simulink model "Furnace"  (R2020a)
settings: Solver=ode15s  StartTime=0  StopTime=27000  FixedStep=0.1  MaxStep=20  MinStep=1e-13  RelTol=1e-08  AbsTol=1e-09
undefined symbols (not defined in the file): agnostic_lqe_params, cont_reg, disturbance_type, F_aI_pid, F_aII_pid, input_type, k, lqe_params, LQR_params, LQRAgnostic_params, MPC_type, MPCDiscrete_function_parameters, MPCDiscreteAgnostic_function_parameters, MPCDiscreteDiffIntegralAgnostic_function_parameters, original_LQR_params, output_type, reg, single_butter_ss
libraries: simulink x35, cstblocks x10, mpclib x3
(part 1 of 8)
settings Model: Creator=elisam  LastModifiedBy=jorn
settings SolverCC: MaxConsecutiveZCs=10000  ZeroCrossAlgorithm=Adaptive
settings DataIOCC: FinalStateName=ss_state_out  InitialState=ss_state  LoadInitialState=on  SaveFinalState=on  SaveOperatingPoint=on  SaveFormat=Array  SaveOutput=off  DSMLogging=off  ReturnWorkspaceOutputs=off
settings OptimizationCC: BlockReduction=off  EfficientMapNaN2IntZero=off  SimCompilerOptimization=on
settings DebuggingCC: AlgebraicLoopMsg=error  ArtificialAlgebraicLoopMsg=error  UnconnectedInputMsg=none  UnconnectedOutputMsg=none  UnconnectedLineMsg=none  PregeneratedLibrarySubsystemCodeDiagnostic=none  ArithmeticOperatorsInVariantConditions=warning
settings HardwareCC: TargetBitPerLong=64  TargetBitPerPointer=64  TargetBitPerSizeT=64  TargetBitPerPtrDiffT=64  TargetLongLongMode=on  TargetIntDivRoundTo=Zero  TargetEndianess=LittleEndian  TargetWordSize=64  TargetHWDeviceType=MATLAB Host  ProdEqTarget=off
settings SFSimCC: SimUseLocalCustomCode=off  CustomCodeUndefinedFunction=UseInterfaceOnly
settings CodeAppCC: MaxIdLength=128
settings GRTTargetCC: CombineOutputUpdateFcns=off  GRTInterface=on

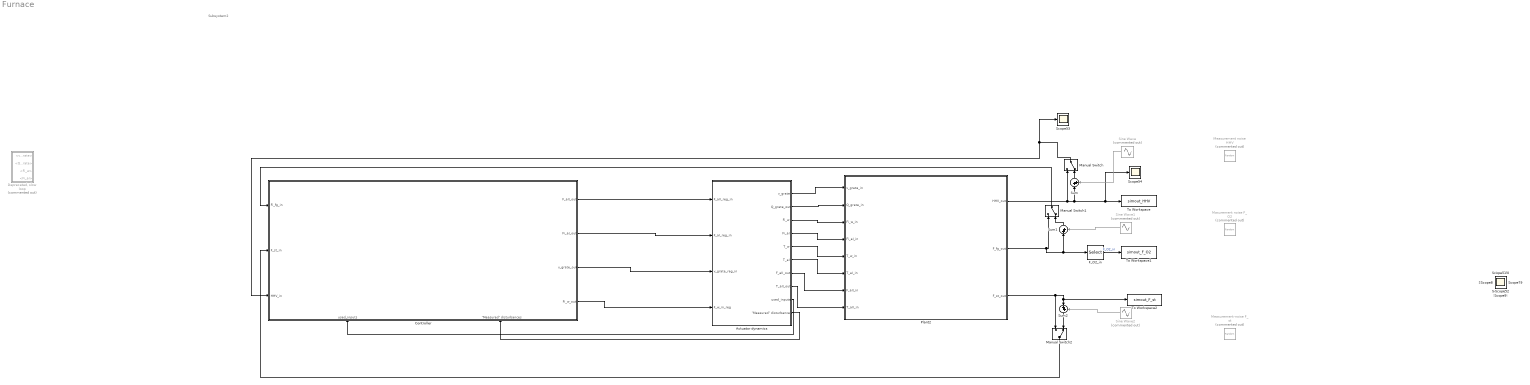
== system Furnace ==
  note: Subsystem2
  Actuator dynamics : Subsystem
  Controller : Subsystem
      settings: PortSchema="{\"entries\":[{\"content\":{\"sides\":[{\"content\":{\"connectorIds\":[\"In1\",\"In2\",\"In3\"]},\"type\":\"ConnectorPlacement.EquallySpacedRectSide\",\"uuid\":\"9212388b-0233-4c0d-abf7-b4aac7804a1a\"},{\"content\":{\"connectorIds\":[\"Out1\",\"Out2\",\"Out3\",\"Out4\"],\"side\":\"RIGHT\"},\"type\":\"ConnectorPlacement.EquallySpacedRectSide\",\"uuid\":\"ec9f57cf-6c7e-4926-bff7-17ce1d99a11a\"},{\"content\":{\"connectorIds\":[],\"side\":\"TOP\"},\"type\":\"ConnectorPlacement.EquallySpacedRectSide\",\"uuid\":\"f3c30994-927b-4377-92d1-6db743f01150\"},{\"content\":{\"connectorIds\":[\"In4\",\"In5\"],\"side\":\"BOTTOM\"},\"type\":\"ConnectorPlacement.EquallySpacedRectSide\",\"uuid\":\"c1a92049-b704-4e72-9e8e-c3f5af65781d\"}]},\"type\":\"ConnectorPlacement.EquallySpacedConnector\",\"uuid\":\"4dfd1ddf-42df-430c-9ebe-da49fca051ac\"}],\"packageUris\":[\"http://schema.mathworks.com/mf0/Connector/19700101\"],\"version\":\"1.0\"}"
  "Deprecated, slow loop" : Subsystem  Commented=on
  F_O2_in : Selector  InputPortWidth=12  IndexOptions=Index vector (dialog)  Indices=[4]  OutputSizes=1
  Manual Switch : ManualSwitch  CurrentSetting=0
  Manual Switch1 : ManualSwitch  CurrentSetting=0
  Manual Switch2 : ManualSwitch  CurrentSetting=0
  Masurement noise F_O2 : RandomNumber  Commented=on  Variance=reg.include_noise*reg.sp_F_O2*1e-3  Seed=2  SampleTime=1
  Measurement noise HHV : RandomNumber  Commented=on  Variance=reg.include_noise*reg.sp_HHV * 1e-3  Seed=1  SampleTime=1
  Measurement-noise F_st : RandomNumber  Commented=on  Variance=reg.include_noise*reg.sp_F_st* 1e-3  Seed=3  SampleTime=1
  Plant2 : Subsystem
  Scope{,1..54} (55 alike) : Scope
  Sine Wave : Sin  Commented=on  Amplitude=reg.include_noise * 1e-3  SampleTime=0
  Sine Wave1 : Sin  Commented=on  Amplitude=reg.include_noise * 1e-3  SampleTime=0
  Sine Wave2 : Sin  Commented=on  Amplitude=reg.include_noise * 1e-3  SampleTime=0
  Sum : Sum  Inputs=|++
  Sum1 : Sum  Inputs=|++
  Sum2 : Sum  Inputs=|++
  To Workspace : ToWorkspace  VariableName=simout_HHV  SaveFormat=Timeseries  SampleTime=-1
  To Workspace1 : ToWorkspace  VariableName=simout_F_O2  SaveFormat=Timeseries  SampleTime=-1
  To Workspace2 : ToWorkspace  VariableName=simout_F_st  SaveFormat=Timeseries  SampleTime=-1
  wires:
  Manual Switch2/1 -> Controller/2(F_st_in)
  Manual Switch/1 -> Scope53/1, Controller/3(HHV_in)
  Manual Switch1/1 -> Controller/1(Fi_fg_in)
  Controller/1(F_aII_out) -> Actuator dynamics/1(F_aII_reg_in)
  Controller/2(Fi_aI_out) -> Actuator dynamics/2("F_aI_reg_in ")
  Controller/3(v_grate_out) -> Actuator dynamics/3(v_grate_reg_in)
  Controller/4(Fi_w_out) -> Actuator dynamics/4(F_w_in_reg)
  Actuator dynamics/1(v_grate) -> Plant2/1(v_grate_in)
  Actuator dynamics/2(Q_grate_out) -> Plant2/2(Q_grate_in)
  Actuator dynamics/3(Fi_w) -> Plant2/3(Fi_w_in)
  Actuator dynamics/4(Fi_aI) -> Plant2/4(Fi_aI_in)
  Actuator dynamics/5(T_w) -> Plant2/5(T_w_in)
  Actuator dynamics/6(T_aI) -> Plant2/6(T_aI_in)
  Actuator dynamics/7(F_aII_out) -> Plant2/7(F_aII_in)
  Actuator dynamics/8(T_aII_out) -> Plant2/8(T_aII_in)
  F_O2_in/1 -> To Workspace1/1  "F_O2_in"
  Actuator dynamics/9(used_inputs) -> Controller/4(used_inputs)
  Sum/1 -> Manual Switch/2
  Plant2/1(HHV_out) -> Manual Switch/1, Scope54/1, To Workspace/1, Sum/1
  Plant2/2(F_fg_out) -> Manual Switch1/1, Sum1/1, F_O2_in/1
  Sum1/1 -> Manual Switch1/2
  Sum2/1 -> Manual Switch2/2
  Plant2/3(F_st_out) -> To Workspace2/1, Sum2/1, Manual Switch2/1
  Sine Wave/1 -> Sum/2
  Sine Wave1/1 -> Sum1/2
  Sine Wave2/1 -> Sum2/2
  Actuator dynamics/10("\"Measured\" disturbances") -> Controller/5("\"Measured\" disturbances")

== system Furnace/Actuator dynamics ==
  F_aII_reg_in : Inport
  "F_aI_reg_in " : Inport  Port=2
  v_grate_reg_in : Inport  Port=3
  F_w_in_reg : Inport  Port=4
  Demux : Demux  Outputs=3
  Grate speed : Subsystem
  Mux : Mux
  Mux1 : Mux  Inputs=5
  Scope : Scope
  Scope1 : Scope
  Scope2 : Scope
  Secondary air : Subsystem
      mask Display: image('airflow.jpeg');
  Waste and Primary air : Subsystem
      mask Display: image('waste_in.jpg');
  v_grate : Outport
  Q_grate_out : Outport  Port=2
  Fi_w : Outport  Port=3
  Fi_aI : Outport  Port=4
  T_w : Outport  Port=5
  T_aI : Outport  Port=6
  F_aII_out : Outport  Port=7
  T_aII_out : Outport  Port=8
  used_inputs : Outport  Port=9
  "\"Measured\" disturbances" : Outport  Port=10
  wires:
  Grate speed/1(v_grate_out) -> v_grate/1  "v_grate"
  Grate speed/2(Q_grate_out) -> Q_grate_out/1, Demux/1
  Secondary air/2(T_aII_out) -> Mux1/2, T_aII_out/1  "T_aII"
  Waste and Primary air/2(Fi_aI_out) -> Fi_aI/1  "Fi_aI"
  Waste and Primary air/3(T_w_out) -> T_w/1  "T_w"
  Waste and Primary air/1(Fi_w_out) -> Fi_w/1  "Fi_w"
  Waste and Primary air/4(T_aI_out) -> Mux1/1, T_aI/1  "T_aI"
  F_w_in_reg/1 -> Waste and Primary air/2(F_w_in_reg)
  Secondary air/1(F_aII_out) -> F_aII_out/1  "F_aII"
  v_grate_reg_in/1 -> Grate speed/1(v_grate_reg_in)
  "F_aI_reg_in "/1 -> Waste and Primary air/1("F_aI_reg_in ")
  F_aII_reg_in/1 -> Secondary air/1(F_aII_reg_in)
  Waste and Primary air/6(u_F_w) -> Mux/4, Scope/1  "u_F_w"
  Waste and Primary air/5(u_Fi_aI) -> Mux/2, Scope1/1  "u_F_aI"
  Secondary air/3(u_F_aII) -> Mux/1, Scope2/1  "u_F_aII"
  Grate speed/3(u_v_grate) -> Mux/3
  Mux/1 -> used_inputs/1
  Mux1/1 -> "\"Measured\" disturbances"/1
  Demux/3 -> Mux1/5
  Demux/2 -> Mux1/4
  Demux/1 -> Mux1/3

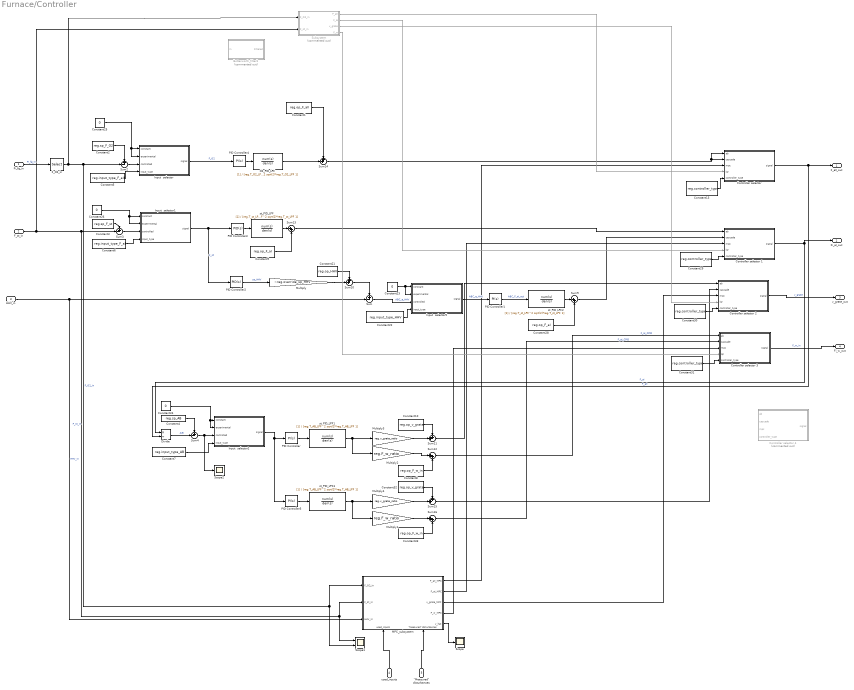
== system Furnace/Controller ==
  Fi_fg_in : Inport
  F_st_in : Inport  Port=2
  HHV_in : Inport  Port=3
  used_inputs : Inport  Port=4
  "\"Measured\" disturbances" : Inport  Port=5
  Butterworth_filter3 : Subsystem  Commented=on
  Constant1 : Constant  Value=reg.op_F_aII
  Constant10 : Constant  Value=reg.op_v_grate
  Constant{13,29..31} (4 alike) : Constant  Value=reg.controller_type
  Constant2 : Constant  Value=reg.sp_F_O2
  Constant21 : Constant  Value=reg.op_HHV
  Constant22 : Constant  Value=reg.input_type_HHV
  Constant{23..26} (4 alike) : Constant  Value=0
  Constant28 : Constant  Value=reg.op_F_aI
  Constant3 : Constant  Value=reg.sp_F_st
  Constant32 : Constant  Value=reg.op_v_grate
  Constant33 : Constant  Value=reg.op_F_w_in
  Constant4 : Constant  Value=reg.sp_AB
  Constant5 : Constant  Value=reg.input_type_F_aII
  Constant6 : Constant  Value=reg.input_type_F_aI
  Constant7 : Constant  Value=reg.input_type_AB
  Constant8 : Constant  Value=reg.op_F_w_in
  Constant9 : Constant  Value=reg.op_F_aI
  "Controller selector " : MATLAB Function  TreatAsAtomicUnit=on
  Controller selector 1 : MATLAB Function  TreatAsAtomicUnit=on
  Controller selector 2 : MATLAB Function  TreatAsAtomicUnit=on
  Controller selector 3 : MATLAB Function  TreatAsAtomicUnit=on
  Controller selector 4 : MATLAB Function  Commented=on  TreatAsAtomicUnit=on
  Divide : Product  Inputs=*/  OutMin=[-100]  OutMax=[100]
  F_O2_in : Selector  InputPortWidth=12  IndexOptions=Index vector (dialog)  Indices=[4]  OutputSizes=1
  Input  selector : MATLAB Function  TreatAsAtomicUnit=on
  Input  selector1 : MATLAB Function  TreatAsAtomicUnit=on
  Input  selector2 : MATLAB Function  TreatAsAtomicUnit=on
  Input  selector5 : MATLAB Function  TreatAsAtomicUnit=on
  MPC_subsystem : Subsystem
      settings: PortSchema="{\"entries\":[{\"content\":{\"sides\":[{\"content\":{\"connectorIds\":[\"In1\",\"In2\",\"In3\"]},\"type\":\"ConnectorPlacement.EquallySpacedRectSide\",\"uuid\":\"7a72dc7f-38c0-42c0-80ed-1e6801fa5538\"},{\"content\":{\"connectorIds\":[\"Out1\",\"Out2\",\"Out3\",\"Out4\",\"Out5\"],\"side\":\"RIGHT\"},\"type\":\"ConnectorPlacement.EquallySpacedRectSide\",\"uuid\":\"3b96338e-56f2-4c6d-b025-d8deebb787e0\"},{\"content\":{\"connectorIds\":[],\"side\":\"TOP\"},\"type\":\"ConnectorPlacement.EquallySpacedRectSide\",\"uuid\":\"204ca672-7e69-45d1-bd78-35e421377db1\"},{\"content\":{\"connectorIds\":[\"In4\",\"In5\"],\"side\":\"BOTTOM\"},\"type\":\"ConnectorPlacement.EquallySpacedRectSide\",\"uuid\":\"d178d855-840b-4794-a5e2-c07226929ecd\"}]},\"type\":\"ConnectorPlacement.EquallySpacedConnector\",\"uuid\":\"1be467ef-13fc-4acb-88f5-eb362f838469\"}],\"packageUris\":[\"http://schema.mathworks.com/mf0/Connector/19700101\"],\"version\":\"1.0\"}"
  Multiply : Gain  Gain=~reg.override_sp_HHV
  Multiply1 : Gain  Gain=reg.F_w_ratio
  Multiply2 : Gain  Gain=reg.F_w_ratio
  Multiply3 : Gain  Gain=reg.v_grate_ratio
  Multiply4 : Gain  Gain=reg.v_grate_ratio
  O2_PID_LPF : TransferFcn  Denominator=[reg.T_O2_LPF^2 sqrt(2)*reg.T_O2_LPF 1]
  PID Controller : simulink/Continuous/PID Controller  Controller=PI  Form=Parallel  TimeDomain=Continuous-time  UseExternalTs=off  SampleTime=1  IntegratorMethod=Forward Euler  FilterMethod=Forward Euler  ControllerParametersSource=internal  P=reg.Kp_AB  I=reg.Ki_AB  D=0  UseFilter=on  N=100  TunerSelectOption=Transfer Function Based (PID Tuner App)  InitialConditionSource=internal  InitialConditionForIntegrator=0  InitialConditionForFilter=0  DifferentiatorICPrevScaledInput=0  ExternalReset=none  TrackingMode=off  Kt=1  LimitOutput=off  UpperSaturationLimit=inf  LowerSaturationLimit=-inf  LinearizeAsGain=on  AntiWindupMode=none  Kb=1  POutMin=[]  POutMax=[]  IOutMin=[]  IOutMax=[]  DOutMin=[]  DOutMax=[]  NOutMin=[]  NOutMax=[]  SumOutMin=[]  SumOutMax=[]  SaturationOutMin=[]  SaturationOutMax=[]  PParamMin=[]  PParamMax=[]  IParamMin=[]  IParamMax=[]  DParamMin=[]  DParamMax=[]  NParamMin=[]  NParamMax=[]  KbParamMin=[]  KbParamMax=[]  KtParamMin=[]  KtParamMax=[]  KbOutMin=[]  KbOutMax=[]  KtOutMin=[]  KtOutMax=[]  IntegratorOutMin=[]  IntegratorOutMax=[]  FilterOutMin=[]  FilterOutMax=[]  SumI1OutMin=[]  SumI1OutMax=[]  SumI2OutMin=[]  SumI2OutMax=[]  SumI3OutMin=[]  SumI3OutMax=[]  SumI4OutMin=[]  SumI4OutMax=[]  SumDOutMin=[]  SumDOutMax=[]  DifferentiatorOutMin=[]  DifferentiatorOutMax=[]  FilterDiffOutCoefMin=[]  FilterDiffOutCoefMax=[]  ReciprocalOutMin=[]  ReciprocalOutMax=[]  SumDenOutMin=[]  SumDenOutMax=[]  SumNumOutMin=[]  SumNumOutMax=[]  DivideOutMin=[]  DivideOutMax=[]  UdiffTsProdOutMin=[]  UdiffTsProdOutMax=[]  NTsProdOutMin=[]  NTsProdOutMax=[]  UintegralTsProdOutMin=[]  UintegralTsProdOutMax=[]  UngainTsProdOutMin=[]  UngainTsProdOutMax=[]  IntegratorContinuousStateAttributes=''  IntegratorStateMustResolveToSignalObject=off  IntegratorRTWStateStorageClass=Auto  FilterContinuousStateAttributes=''  FilterStateMustResolveToSignalObject=off  FilterRTWStateStorageClass=Auto  ParallelPVariant=InternalParameters  IdealPVariant=Disabled  IVariant=InternalParameters  DVariant=Disabled  IntegratorVariant=Continuous  SatVariant=Disabled  AWVariant=Passthrough  PCopyVariant=Disabled  TRVariant=Disabled  FdbkBlocksVariant=Forward  IdealPFdbkVariant=Disabled  SatFdbkVariant=Disabled  DerivativeFilterVariant=Disabled  NVariant=Disabled  NCopyVariant=Disabled_SignalSpec  FilterICVariant=Disabled  IntegratorICVariant=InternalICs  ExternalResetVariant=Disabled  TRSumVariant=Passthrough  SumFdbkVariant=Disabled  SumVariant=Sum_PI  TsampFilterVariant=InternalTs  TsampNgainVariant=Passthrough  TsampIntegralVariant=Passthrough
  PID Controller1 : simulink/Continuous/PID Controller  Controller=PI  Form=Parallel  TimeDomain=Continuous-time  UseExternalTs=off  SampleTime=1  IntegratorMethod=Forward Euler  FilterMethod=Forward Euler  ControllerParametersSource=internal  P=reg.Kp_HHV  I=reg.Ki_HHV  D=0  UseFilter=on  N=100  TunerSelectOption=Transfer Function Based (PID Tuner App)  InitialConditionSource=internal  InitialConditionForIntegrator=0  InitialConditionForFilter=0  DifferentiatorICPrevScaledInput=0  ExternalReset=none  TrackingMode=off  Kt=1  LimitOutput=off  UpperSaturationLimit=inf  LowerSaturationLimit=-inf  LinearizeAsGain=on  AntiWindupMode=none  Kb=1  POutMin=[]  POutMax=[]  IOutMin=[]  IOutMax=[]  DOutMin=[]  DOutMax=[]  NOutMin=[]  NOutMax=[]  SumOutMin=[]  SumOutMax=[]  SaturationOutMin=[]  SaturationOutMax=[]  PParamMin=[]  PParamMax=[]  IParamMin=[]  IParamMax=[]  DParamMin=[]  DParamMax=[]  NParamMin=[]  NParamMax=[]  KbParamMin=[]  KbParamMax=[]  KtParamMin=[]  KtParamMax=[]  KbOutMin=[]  KbOutMax=[]  KtOutMin=[]  KtOutMax=[]  IntegratorOutMin=[]  IntegratorOutMax=[]  FilterOutMin=[]  FilterOutMax=[]  SumI1OutMin=[]  SumI1OutMax=[]  SumI2OutMin=[]  SumI2OutMax=[]  SumI3OutMin=[]  SumI3OutMax=[]  SumI4OutMin=[]  SumI4OutMax=[]  SumDOutMin=[]  SumDOutMax=[]  DifferentiatorOutMin=[]  DifferentiatorOutMax=[]  FilterDiffOutCoefMin=[]  FilterDiffOutCoefMax=[]  ReciprocalOutMin=[]  ReciprocalOutMax=[]  SumDenOutMin=[]  SumDenOutMax=[]  SumNumOutMin=[]  SumNumOutMax=[]  DivideOutMin=[]  DivideOutMax=[]  UdiffTsProdOutMin=[]  UdiffTsProdOutMax=[]  NTsProdOutMin=[]  NTsProdOutMax=[]  UintegralTsProdOutMin=[]  UintegralTsProdOutMax=[]  UngainTsProdOutMin=[]  UngainTsProdOutMax=[]  IntegratorContinuousStateAttributes=''  IntegratorStateMustResolveToSignalObject=off  IntegratorRTWStateStorageClass=Auto  FilterContinuousStateAttributes=''  FilterStateMustResolveToSignalObject=off  FilterRTWStateStorageClass=Auto  ParallelPVariant=InternalParameters  IdealPVariant=Disabled  IVariant=InternalParameters  DVariant=Disabled  IntegratorVariant=Continuous  SatVariant=Disabled  AWVariant=Passthrough  PCopyVariant=Disabled  TRVariant=Disabled  FdbkBlocksVariant=Forward  IdealPFdbkVariant=Disabled  SatFdbkVariant=Disabled  DerivativeFilterVariant=Disabled  NVariant=Disabled  NCopyVariant=Disabled_SignalSpec  FilterICVariant=Disabled  IntegratorICVariant=InternalICs  ExternalResetVariant=Disabled  TRSumVariant=Passthrough  SumFdbkVariant=Disabled  SumVariant=Sum_PI  TsampFilterVariant=InternalTs  TsampNgainVariant=Passthrough  TsampIntegralVariant=Passthrough
  PID Controller2 : simulink/Continuous/PID Controller  Controller=PID  Form=Parallel  TimeDomain=Continuous-time  UseExternalTs=off  SampleTime=1  IntegratorMethod=Forward Euler  FilterMethod=Forward Euler  ControllerParametersSource=internal  P=reg.Kp_st_HHV  I=reg.Ki_st_HHV  D=reg.Kd_st_HHV  UseFilter=on  N=100  TunerSelectOption=Transfer Function Based (PID Tuner App)  InitialConditionSource=internal  InitialConditionForIntegrator=0.001  InitialConditionForFilter=0  DifferentiatorICPrevScaledInput=0  ExternalReset=none  TrackingMode=off  Kt=1  LimitOutput=off  UpperSaturationLimit=inf  LowerSaturationLimit=1  LinearizeAsGain=on  AntiWindupMode=none  Kb=1  POutMin=[]  POutMax=[]  IOutMin=[]  IOutMax=[]  DOutMin=[]  DOutMax=[]  NOutMin=[]  NOutMax=[]  SumOutMin=[]  SumOutMax=[]  SaturationOutMin=[]  SaturationOutMax=[]  PParamMin=[]  PParamMax=[]  IParamMin=[]  IParamMax=[]  DParamMin=[]  DParamMax=[]  NParamMin=[]  NParamMax=[]  KbParamMin=[]  KbParamMax=[]  KtParamMin=[]  KtParamMax=[]  KbOutMin=[]  KbOutMax=[]  KtOutMin=[]  KtOutMax=[]  IntegratorOutMin=[]  IntegratorOutMax=[]  FilterOutMin=[]  FilterOutMax=[]  SumI1OutMin=[]  SumI1OutMax=[]  SumI2OutMin=[]  SumI2OutMax=[]  SumI3OutMin=[]  SumI3OutMax=[]  SumI4OutMin=[]  SumI4OutMax=[]  SumDOutMin=[]  SumDOutMax=[]  DifferentiatorOutMin=[]  DifferentiatorOutMax=[]  FilterDiffOutCoefMin=[]  FilterDiffOutCoefMax=[]  ReciprocalOutMin=[]  ReciprocalOutMax=[]  SumDenOutMin=[]  SumDenOutMax=[]  SumNumOutMin=[]  SumNumOutMax=[]  DivideOutMin=[]  DivideOutMax=[]  UdiffTsProdOutMin=[]  UdiffTsProdOutMax=[]  NTsProdOutMin=[]  NTsProdOutMax=[]  UintegralTsProdOutMin=[]  UintegralTsProdOutMax=[]  UngainTsProdOutMin=[]  UngainTsProdOutMax=[]  IntegratorContinuousStateAttributes='F_st'  IntegratorStateMustResolveToSignalObject=off  IntegratorRTWStateStorageClass=Auto  FilterContinuousStateAttributes=''  FilterStateMustResolveToSignalObject=off  FilterRTWStateStorageClass=Auto  ParallelPVariant=InternalParameters  IdealPVariant=Disabled  IVariant=InternalParameters  DVariant=InternalParameters  IntegratorVariant=Continuous  SatVariant=Disabled  AWVariant=Passthrough  PCopyVariant=Disabled  TRVariant=Disabled  FdbkBlocksVariant=Forward  IdealPFdbkVariant=Disabled  SatFdbkVariant=Disabled  DerivativeFilterVariant=ContFilter  NVariant=InternalParameters  NCopyVariant=Disabled  FilterICVariant=InternalICsFilter  IntegratorICVariant=InternalICs  ExternalResetVariant=Disabled  TRSumVariant=Passthrough  SumFdbkVariant=Disabled  SumVariant=Sum_PID  TsampFilterVariant=InternalTs  TsampNgainVariant=Passthrough  TsampIntegralVariant=Passthrough
  PID Controller3 : simulink/Continuous/PID Controller  Controller=PID  Form=Parallel  TimeDomain=Continuous-time  UseExternalTs=off  SampleTime=1  IntegratorMethod=Forward Euler  FilterMethod=Forward Euler  ControllerParametersSource=internal  P=reg.Kp_st  I=reg.Ki_st  D=reg.Kd_st  UseFilter=on  N=100  TunerSelectOption=Transfer Function Based (PID Tuner App)  InitialConditionSource=internal  InitialConditionForIntegrator=0  InitialConditionForFilter=0  DifferentiatorICPrevScaledInput=0  ExternalReset=none  TrackingMode=off  Kt=1  LimitOutput=off  UpperSaturationLimit=inf  LowerSaturationLimit=1  LinearizeAsGain=on  AntiWindupMode=none  Kb=1  POutMin=[]  POutMax=[]  IOutMin=[]  IOutMax=[]  DOutMin=[]  DOutMax=[]  NOutMin=[]  NOutMax=[]  SumOutMin=[]  SumOutMax=[]  SaturationOutMin=[]  SaturationOutMax=[]  PParamMin=[]  PParamMax=[]  IParamMin=[]  IParamMax=[]  DParamMin=[]  DParamMax=[]  NParamMin=[]  NParamMax=[]  KbParamMin=[]  KbParamMax=[]  KtParamMin=[]  KtParamMax=[]  KbOutMin=[]  KbOutMax=[]  KtOutMin=[]  KtOutMax=[]  IntegratorOutMin=[]  IntegratorOutMax=[]  FilterOutMin=[]  FilterOutMax=[]  SumI1OutMin=[]  SumI1OutMax=[]  SumI2OutMin=[]  SumI2OutMax=[]  SumI3OutMin=[]  SumI3OutMax=[]  SumI4OutMin=[]  SumI4OutMax=[]  SumDOutMin=[]  SumDOutMax=[]  DifferentiatorOutMin=[]  DifferentiatorOutMax=[]  FilterDiffOutCoefMin=[]  FilterDiffOutCoefMax=[]  ReciprocalOutMin=[]  ReciprocalOutMax=[]  SumDenOutMin=[]  SumDenOutMax=[]  SumNumOutMin=[]  SumNumOutMax=[]  DivideOutMin=[]  DivideOutMax=[]  UdiffTsProdOutMin=[]  UdiffTsProdOutMax=[]  NTsProdOutMin=[]  NTsProdOutMax=[]  UintegralTsProdOutMin=[]  UintegralTsProdOutMax=[]  UngainTsProdOutMin=[]  UngainTsProdOutMax=[]  IntegratorContinuousStateAttributes='F_st'  IntegratorStateMustResolveToSignalObject=off  IntegratorRTWStateStorageClass=Auto  FilterContinuousStateAttributes=''  FilterStateMustResolveToSignalObject=off  FilterRTWStateStorageClass=Auto  ParallelPVariant=InternalParameters  IdealPVariant=Disabled  IVariant=InternalParameters  DVariant=InternalParameters  IntegratorVariant=Continuous  SatVariant=Disabled  AWVariant=Passthrough  PCopyVariant=Disabled  TRVariant=Disabled  FdbkBlocksVariant=Forward  IdealPFdbkVariant=Disabled  SatFdbkVariant=Disabled  DerivativeFilterVariant=ContFilter  NVariant=InternalParameters  NCopyVariant=Disabled  FilterICVariant=InternalICsFilter  IntegratorICVariant=InternalICs  ExternalResetVariant=Disabled  TRSumVariant=Passthrough  SumFdbkVariant=Disabled  SumVariant=Sum_PID  TsampFilterVariant=InternalTs  TsampNgainVariant=Passthrough  TsampIntegralVariant=Passthrough
  PID Controller4 : simulink/Continuous/PID Controller  Controller=PI  Form=Parallel  TimeDomain=Continuous-time  UseExternalTs=off  SampleTime=1  IntegratorMethod=Forward Euler  FilterMethod=Forward Euler  ControllerParametersSource=internal  P=reg.Kp_O2  I=reg.Ki_O2  D=0  UseFilter=on  N=100  TunerSelectOption=Transfer Function Based (PID Tuner App)  InitialConditionSource=internal  InitialConditionForIntegrator=0.001  InitialConditionForFilter=0  DifferentiatorICPrevScaledInput=0  ExternalReset=none  TrackingMode=off  Kt=1  LimitOutput=off  UpperSaturationLimit=inf  LowerSaturationLimit=1  LinearizeAsGain=on  AntiWindupMode=none  Kb=1  POutMin=[]  POutMax=[]  IOutMin=[]  IOutMax=[]  DOutMin=[]  DOutMax=[]  NOutMin=[]  NOutMax=[]  SumOutMin=[]  SumOutMax=[]  SaturationOutMin=[]  SaturationOutMax=[]  PParamMin=[]  PParamMax=[]  IParamMin=[]  IParamMax=[]  DParamMin=[]  DParamMax=[]  NParamMin=[]  NParamMax=[]  KbParamMin=[]  KbParamMax=[]  KtParamMin=[]  KtParamMax=[]  KbOutMin=[]  KbOutMax=[]  KtOutMin=[]  KtOutMax=[]  IntegratorOutMin=[]  IntegratorOutMax=[]  FilterOutMin=[]  FilterOutMax=[]  SumI1OutMin=[]  SumI1OutMax=[]  SumI2OutMin=[]  SumI2OutMax=[]  SumI3OutMin=[]  SumI3OutMax=[]  SumI4OutMin=[]  SumI4OutMax=[]  SumDOutMin=[]  SumDOutMax=[]  DifferentiatorOutMin=[]  DifferentiatorOutMax=[]  FilterDiffOutCoefMin=[]  FilterDiffOutCoefMax=[]  ReciprocalOutMin=[]  ReciprocalOutMax=[]  SumDenOutMin=[]  SumDenOutMax=[]  SumNumOutMin=[]  SumNumOutMax=[]  DivideOutMin=[]  DivideOutMax=[]  UdiffTsProdOutMin=[]  UdiffTsProdOutMax=[]  NTsProdOutMin=[]  NTsProdOutMax=[]  UintegralTsProdOutMin=[]  UintegralTsProdOutMax=[]  UngainTsProdOutMin=[]  UngainTsProdOutMax=[]  IntegratorContinuousStateAttributes='F_st'  IntegratorStateMustResolveToSignalObject=off  IntegratorRTWStateStorageClass=Auto  FilterContinuousStateAttributes=''  FilterStateMustResolveToSignalObject=off  FilterRTWStateStorageClass=Auto  ParallelPVariant=InternalParameters  IdealPVariant=Disabled  IVariant=InternalParameters  DVariant=Disabled  IntegratorVariant=Continuous  SatVariant=Disabled  AWVariant=Passthrough  PCopyVariant=Disabled  TRVariant=Disabled  FdbkBlocksVariant=Forward  IdealPFdbkVariant=Disabled  SatFdbkVariant=Disabled  DerivativeFilterVariant=Disabled  NVariant=Disabled  NCopyVariant=Disabled_SignalSpec  FilterICVariant=Disabled  IntegratorICVariant=InternalICs  ExternalResetVariant=Disabled  TRSumVariant=Passthrough  SumFdbkVariant=Disabled  SumVariant=Sum_PI  TsampFilterVariant=InternalTs  TsampNgainVariant=Passthrough  TsampIntegralVariant=Passthrough
  PID Controller5 : simulink/Continuous/PID Controller  Controller=PI  Form=Parallel  TimeDomain=Continuous-time  UseExternalTs=off  SampleTime=1  IntegratorMethod=Forward Euler  FilterMethod=Forward Euler  ControllerParametersSource=internal  P=reg.Kp_AB_HHV  I=reg.Ki_AB_HHV  D=0  UseFilter=on  N=100  TunerSelectOption=Transfer Function Based (PID Tuner App)  InitialConditionSource=internal  InitialConditionForIntegrator=0  InitialConditionForFilter=0  DifferentiatorICPrevScaledInput=0  ExternalReset=none  TrackingMode=off  Kt=1  LimitOutput=off  UpperSaturationLimit=inf  LowerSaturationLimit=-inf  LinearizeAsGain=on  AntiWindupMode=none  Kb=1  POutMin=[]  POutMax=[]  IOutMin=[]  IOutMax=[]  DOutMin=[]  DOutMax=[]  NOutMin=[]  NOutMax=[]  SumOutMin=[]  SumOutMax=[]  SaturationOutMin=[]  SaturationOutMax=[]  PParamMin=[]  PParamMax=[]  IParamMin=[]  IParamMax=[]  DParamMin=[]  DParamMax=[]  NParamMin=[]  NParamMax=[]  KbParamMin=[]  KbParamMax=[]  KtParamMin=[]  KtParamMax=[]  KbOutMin=[]  KbOutMax=[]  KtOutMin=[]  KtOutMax=[]  IntegratorOutMin=[]  IntegratorOutMax=[]  FilterOutMin=[]  FilterOutMax=[]  SumI1OutMin=[]  SumI1OutMax=[]  SumI2OutMin=[]  SumI2OutMax=[]  SumI3OutMin=[]  SumI3OutMax=[]  SumI4OutMin=[]  SumI4OutMax=[]  SumDOutMin=[]  SumDOutMax=[]  DifferentiatorOutMin=[]  DifferentiatorOutMax=[]  FilterDiffOutCoefMin=[]  FilterDiffOutCoefMax=[]  ReciprocalOutMin=[]  ReciprocalOutMax=[]  SumDenOutMin=[]  SumDenOutMax=[]  SumNumOutMin=[]  SumNumOutMax=[]  DivideOutMin=[]  DivideOutMax=[]  UdiffTsProdOutMin=[]  UdiffTsProdOutMax=[]  NTsProdOutMin=[]  NTsProdOutMax=[]  UintegralTsProdOutMin=[]  UintegralTsProdOutMax=[]  UngainTsProdOutMin=[]  UngainTsProdOutMax=[]  IntegratorContinuousStateAttributes=''  IntegratorStateMustResolveToSignalObject=off  IntegratorRTWStateStorageClass=Auto  FilterContinuousStateAttributes=''  FilterStateMustResolveToSignalObject=off  FilterRTWStateStorageClass=Auto  ParallelPVariant=InternalParameters  IdealPVariant=Disabled  IVariant=InternalParameters  DVariant=Disabled  IntegratorVariant=Continuous  SatVariant=Disabled  AWVariant=Passthrough  PCopyVariant=Disabled  TRVariant=Disabled  FdbkBlocksVariant=Forward  IdealPFdbkVariant=Disabled  SatFdbkVariant=Disabled  DerivativeFilterVariant=Disabled  NVariant=Disabled  NCopyVariant=Disabled_SignalSpec  FilterICVariant=Disabled  IntegratorICVariant=InternalICs  ExternalResetVariant=Disabled  TRSumVariant=Passthrough  SumFdbkVariant=Disabled  SumVariant=Sum_PI  TsampFilterVariant=InternalTs  TsampNgainVariant=Passthrough  TsampIntegralVariant=Passthrough
  Scope : Scope
  Scope1 : Scope  NumInputPorts=2
  Scope2 : Scope
  Subsystem : Subsystem  Commented=on
  Sum{,2..4} (4 alike) : Sum  Inputs=+-|
  Sum{10..11,14..15} (4 alike) : Sum  Inputs=++|
  Sum{9,12..13,16} (4 alike) : Sum  Inputs=|++
  st_PID_LPF : TransferFcn  Denominator=[reg.T_st_LPF^2 sqrt(2)*reg.T_st_LPF 1]
  st_PID_LPF1 : TransferFcn  Denominator=[reg.T_AB_LPF^2 sqrt(2)*reg.T_AB_LPF 1]
  st_PID_LPF2 : TransferFcn  Denominator=[reg.T_st_LPF^2 sqrt(2)*reg.T_st_LPF 1]
  st_PID_LPF3 : TransferFcn  Denominator=[reg.T_AB_LPF^2 sqrt(2)*reg.T_AB_LPF 1]
  F_aII_out : Outport  VectorParamsAs1DForOutWhenUnconnected=off
  Fi_aI_out : Outport  Port=2  VectorParamsAs1DForOutWhenUnconnected=off
  v_grate_out : Outport  Port=3  VectorParamsAs1DForOutWhenUnconnected=off
  Fi_w_out : Outport  Port=4  VectorParamsAs1DForOutWhenUnconnected=off
  wires:
  Input  selector/1(signal) -> PID Controller4/1  "F_O2"
  Constant7/1 -> Input  selector2/4(input_type)
  Constant5/1 -> Input  selector/4(input_type)
  Constant4/1 -> Sum4/1
  Fi_fg_in/1 -> F_O2_in/1  "Fi_fg_in"
  Constant2/1 -> Sum2/1
  F_st_in/1 -> Subsystem/2(F_st_in), Scope1/1, MPC_subsystem/2(F_st_in), Sum3/2  "F_st_in"
  Constant3/1 -> Sum3/1
  F_O2_in/1 -> Subsystem/1(F_O2_in), Scope1/2, MPC_subsystem/1(F_O2_in), Sum2/2  "F_O2_in"
  PID Controller4/1 -> O2_PID_LPF/1
  Sum14/1 -> "Controller selector "/1(ab), "Controller selector "/2(cascade)
  PID Controller3/1 -> st_PID_LPF/1
  Sum13/1 -> Controller selector 1/1(ab)
  Constant8/1 -> Sum12/2
  PID Controller/1 -> st_PID_LPF1/1
  Sum11/1 -> Controller selector 2/1(ab)
  Multiply2/1 -> Sum12/1
  Constant10/1 -> Sum11/1
  st_PID_LPF/1 -> Sum13/1
  st_PID_LPF1/1 -> Multiply2/1, Multiply3/1
  "Controller selector "/1(signal) -> Divide/2, F_aII_out/1  "F_aII"
  Controller selector 1/1(signal) -> Fi_aI_out/1, Divide/1  "F_aI"
  Controller selector 2/1(signal) -> v_grate_out/1  "v_grate"
  Controller selector 3/1(signal) -> Fi_w_out/1  "F_w_in"
  HHV_in/1 -> MPC_subsystem/3(HHV_in), Sum/2  "HHV_in"
  Input  selector5/1(signal) -> PID Controller1/1  "ABC_e_HHV"
  Constant22/1 -> Input  selector5/4(input_type)
  Sum/1 -> Input  selector5/3(controlled)  "ABC_e_HHV"
  Constant23/1 -> Input  selector5/2(experimental), Input  selector5/1(constant)
  Divide/1 -> Sum4/2  "A/B"
  Sum4/1 -> Scope2/1, Input  selector2/3(controlled)
  Input  selector2/1(signal) -> PID Controller5/1, PID Controller/1
  Constant24/1 -> Input  selector2/2(experimental), Input  selector2/1(constant)
  Sum2/1 -> Input  selector/3(controlled)
  Constant25/1 -> Input  selector/2(experimental), Input  selector/1(constant)
  Sum3/1 -> Input  selector1/3(controlled)
  Constant6/1 -> Input  selector1/4(input_type)
  Constant26/1 -> Input  selector1/2(experimental), Input  selector1/1(constant)
  Input  selector1/1(signal) -> PID Controller3/1, PID Controller2/1  "F_st"
  Sum12/1 -> Controller selector 3/1(ab)  "F_aI_CPID"
  PID Controller1/1 -> st_PID_LPF2/1  "ABC_F_aI_out"
  Sum9/1 -> Controller selector 1/2(cascade)
  PID Controller2/1 -> Multiply/1  "sp_HHV"
  Multiply/1 -> Sum10/2
  Constant21/1 -> Sum10/1
  Sum10/1 -> Sum/1
  st_PID_LPF2/1 -> Sum9/1
  Constant28/1 -> Sum9/2
  Constant9/1 -> Sum13/2
  O2_PID_LPF/1 -> Sum14/2
  Constant1/1 -> Sum14/1
  Constant13/1 -> "Controller selector "/5(controller_type)
  Constant29/1 -> Controller selector 1/5(controller_type)
  Constant30/1 -> Controller selector 2/5(controller_type)
  Constant31/1 -> Controller selector 3/5(controller_type)
  st_PID_LPF3/1 -> Multiply1/1, Multiply4/1
  PID Controller5/1 -> st_PID_LPF3/1
  Constant33/1 -> Sum16/2
  Constant32/1 -> Sum15/1
  Multiply1/1 -> Sum16/1
  Sum15/1 -> Controller selector 2/2(cascade)
  Sum16/1 -> Controller selector 3/2(cascade)  "F_aI_CPID"
  Multiply3/1 -> Sum11/2
  Multiply4/1 -> Sum15/2
  MPC_subsystem/1(F_aII_MPC) -> "Controller selector "/3(mpc)
  MPC_subsystem/2(F_aI_MPC) -> Controller selector 1/3(mpc)
  MPC_subsystem/3(v_grate_MPC) -> Controller selector 2/3(mpc)
  MPC_subsystem/4(F_w_MPC) -> Controller selector 3/3(mpc)
  MPC_subsystem/5(y_hat) -> Scope/1
  used_inputs/1 -> MPC_subsystem/4(used_inputs)
  "\"Measured\" disturbances"/1 -> MPC_subsystem/5("\"Measured\" disturbances")
  Subsystem/1(F_aII) -> "Controller selector "/4(lqr)
  Subsystem/2(F_aI) -> Controller selector 1/4(lqr)
  Subsystem/3(v_grate) -> Controller selector 2/4(lqr)
  Subsystem/4(F_w) -> Controller selector 3/4(lqr)

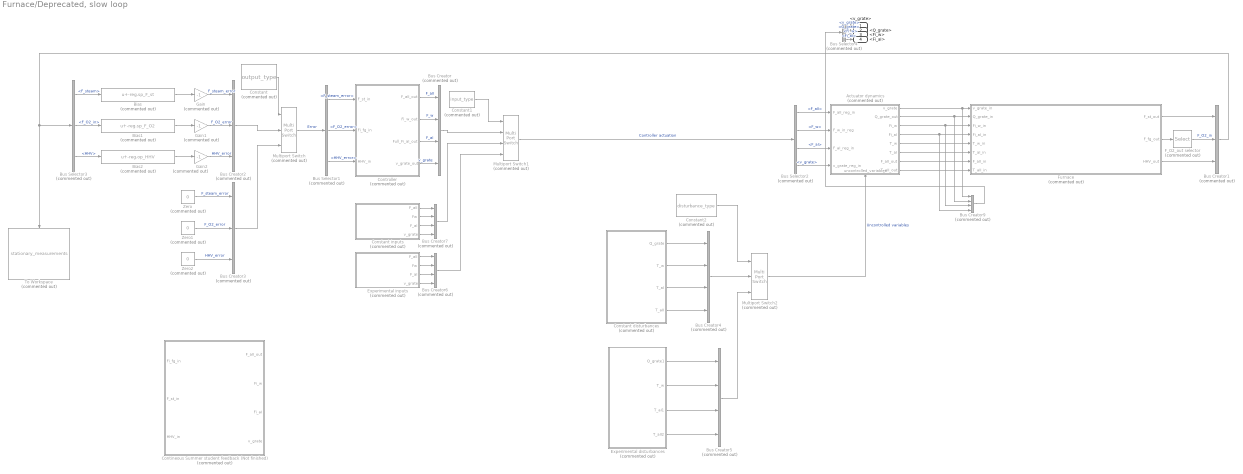
== system Furnace/Deprecated, slow loop ==
  Actuator dynamics : Subsystem  Commented=on
      settings: PortSchema="{\"entries\":[{\"content\":{\"sides\":[{\"content\":{\"connectorIds\":[\"In1\",\"In2\",\"In3\",\"In4\"]},\"type\":\"ConnectorPlacement.EquallySpacedRectSide\",\"uuid\":\"9c70279c-77f9-448c-8401-2f06341e8012\"},{\"content\":{\"connectorIds\":[\"Out1\",\"Out2\",\"Out3\",\"Out4\",\"Out5\",\"Out6\",\"Out7\",\"Out8\"],\"side\":\"RIGHT\"},\"type\":\"ConnectorPlacement.EquallySpacedRectSide\",\"uuid\":\"0d335fa3-f4dc-4bda-8bf3-a847576543d6\"},{\"content\":{\"connectorIds\":[],\"side\":\"TOP\"},\"type\":\"ConnectorPlacement.EquallySpacedRectSide\",\"uuid\":\"42443c55-e82b-4a0c-ba39-8dc1b4207432\"},{\"content\":{\"connectorIds\":[\"In5\"],\"side\":\"BOTTOM\"},\"type\":\"ConnectorPlacement.EquallySpacedRectSide\",\"uuid\":\"9a9600f9-c057-4c7d-b623-b488de804331\"}]},\"type\":\"ConnectorPlacement.EquallySpacedConnector\",\"uuid\":\"1cd21417-d31a-45f7-8451-4b83017cbc67\"}],\"packageUris\":[\"http://schema.mathworks.com/mf0/Connector/19700101\"],\"version\":\"1.0\"}"
  Bias : Bias  Commented=on  Bias=-reg.sp_F_st
  Bias1 : Bias  Commented=on  Bias=-reg.sp_F_O2
  Bias2 : Bias  Commented=on  Bias=-reg.op_HHV
  Bus Creator{,4..7,9} (6 alike) : BusCreator  Commented=on  Inputs=4
  Bus Creator1 : BusCreator  Commented=on  Inputs=3
  Bus Creator2 : BusCreator  Commented=on  Inputs=3
  Bus Creator3 : BusCreator  Commented=on  Inputs=3
  Bus Selector1 : BusSelector  Commented=on  OutputSignals=F_steam_error,F_O2_error,HHV_error
  Bus Selector2 : BusSelector  Commented=on  OutputSignals=F_aII,F_w,F_aI,v_grate
  Bus Selector3 : BusSelector  Commented=on  OutputSignals=F_steam,F_O2_in,HHV
  Bus Selector4 : BusSelector  Commented=on  OutputSignals=v_grate,Q_grate,Fi_w,Fi_aI
  Constant : Constant  Commented=on  Value=output_type
  Constant disturbances : Subsystem  Commented=on
  Constant inputs : Subsystem  Commented=on
  Constant1 : Constant  Commented=on  Value=input_type
  Constant2 : Constant  Commented=on  Value=disturbance_type
  Contineous Summer student feedback (Not finished) : Subsystem  Commented=on
  Controller : Subsystem  Commented=on
  Experimental disturbances : Subsystem  Commented=on
  Experimental inputs : Subsystem  Commented=on
  F_O2_out selector : Selector  Commented=on  InputPortWidth=12  IndexOptions=Index vector (dialog)  Indices=[4]  OutputSizes=1
  Furnace : Subsystem  Commented=on
  Gain : Gain  Commented=on  Gain=-1
  Gain1 : Gain  Commented=on  Gain=-1
  Gain2 : Gain  Commented=on  Gain=-1
  Multiport Switch : MultiPortSwitch  Commented=on  Inputs=2
  Multiport Switch1 : MultiPortSwitch  Commented=on
  Multiport Switch2 : MultiPortSwitch  Commented=on  Inputs=2
  To Workspace : ToWorkspace  Commented=on  VariableName=stationary_measurements  SaveFormat=Timeseries  SampleTime=-1
      settings: MaxDataPoints=1
  Zero : Constant  Commented=on  Value=0  OutDataTypeStr=Inherit: Inherit via back propagation
  Zero1 : Constant  Commented=on  Value=0  OutDataTypeStr=Inherit: Inherit via back propagation
  Zero2 : Constant  Commented=on  Value=0  OutDataTypeStr=Inherit: Inherit via back propagation
  <v_grate> : Outport
  <Q_grate> : Outport  Port=2
  <Fi_w> : Outport  Port=3
  <Fi_aI> : Outport  Port=4
  wires:
  Bus Selector2/2 -> Actuator dynamics/2(F_w_in_reg)  "<F_w>"
  Actuator dynamics/5(T_w) -> Furnace/5(T_w_in)
  Actuator dynamics/6(T_aI) -> Furnace/6(T_aI_in)
  Experimental disturbances/1(Q_grate1) -> Bus Creator5/1
  Actuator dynamics/7(F_aII_out) -> Furnace/7(F_aII_in)
  Furnace/1(F_st_out) -> Bus Creator1/1
  Experimental disturbances/3(T_aI1) -> Bus Creator5/3
  Experimental disturbances/4(T_aII2) -> Bus Creator5/4
  Actuator dynamics/4(Fi_aI) -> Bus Creator9/4, Furnace/4(Fi_aI_in)
  Multiport Switch2/1 -> Actuator dynamics/5(uncontrolled_variables)  "Uncontrolled variables"
  Experimental inputs/2(Fw) -> Bus Creator6/2
  Bus Creator9/1 -> Bus Selector4/1
  Constant inputs/4(v_grate) -> Bus Creator7/4
  Bus Creator2/1 -> Multiport Switch/2
  Controller/1(F_aII_out) -> Bus Creator/1  "F_aII"
  Constant1/1 -> Multiport Switch1/1
  Bus Creator1/1 -> To Workspace/1, Bus Selector3/1
  Actuator dynamics/2(Q_grate_out) -> Bus Creator9/2, Furnace/2(Q_grate_in)
  Furnace/2(F_fg_out) -> F_O2_out selector/1
  Bus Selector3/2 -> Bias1/1  "<F_O2_in>"
  Constant disturbances/2(T_w) -> Bus Creator4/2
  Constant/1 -> Multiport Switch/1
  Bus Selector2/3 -> Actuator dynamics/3("F_aI_reg_in ")  "<F_aI>"
  Bus Selector1/3 -> Controller/3(HHV_in)  "<HHV_error>"
  Constant disturbances/3(T_aI) -> Bus Creator4/3
  Constant disturbances/4(T_aII) -> Bus Creator4/4
  Bus Selector1/2 -> Controller/2(Fi_fg_in)  "<F_O2_error>"
  Experimental inputs/4(v_grate) -> Bus Creator6/4
  Constant disturbances/1(Q_grate) -> Bus Creator4/1
  Constant inputs/1(F_aII) -> Bus Creator7/1
  Furnace/3(HHV_out) -> Bus Creator1/3
  Bus Selector2/4 -> Actuator dynamics/4(v_grate_reg_in)  "<v_grate>"
  Gain/1 -> Bus Creator2/1  "F_steam_error"
  Controller/2(Fi_w_out) -> Bus Creator/2  "F_w"
  Controller/3(Full_Fi_aI_out) -> Bus Creator/3  "F_aI"
  F_O2_out selector/1 -> Bus Creator1/2  "F_O2_in"
  Actuator dynamics/1(v_grate) -> Bus Creator9/1, Furnace/1(v_grate_in)
  Bus Creator5/1 -> Multiport Switch2/3
  Bias1/1 -> Gain1/1
  Controller/4(v_grate_out) -> Bus Creator/4  "v_grate"
  Experimental inputs/3(F_aI) -> Bus Creator6/3
  Multiport Switch1/1 -> Bus Selector2/1  "Controller actuation"
  Bias/1 -> Gain/1
  Bus Selector1/1 -> Controller/1(F_st_in)  "<F_steam_error>"
  Gain2/1 -> Bus Creator2/3  "HHV_error"
  Multiport Switch/1 -> Bus Selector1/1  "Error"
  Bus Creator7/1 -> Multiport Switch1/3
  Bus Selector3/1 -> Bias/1  "<F_steam>"
  Actuator dynamics/3(Fi_w) -> Bus Creator9/3, Furnace/3(Fi_w_in)
  Zero/1 -> Bus Creator3/1  "F_steam_error"
  Experimental inputs/1(F_aII) -> Bus Creator6/1
  Bus Creator/1 -> Multiport Switch1/2
  Bus Creator3/1 -> Multiport Switch/3
  Bus Selector3/3 -> Bias2/1  "<HHV>"
  Constant2/1 -> Multiport Switch2/1
  Bus Creator6/1 -> Multiport Switch1/4
  Experimental disturbances/2(T_w) -> Bus Creator5/2
  Zero1/1 -> Bus Creator3/2  "F_O2_error"
  Bus Selector2/1 -> Actuator dynamics/1(F_aII_reg_in)  "<F_aII>"
  Bias2/1 -> Gain2/1
  Zero2/1 -> Bus Creator3/3  "HHV_error"
  Gain1/1 -> Bus Creator2/2  "F_O2_error"
  Actuator dynamics/8(T_aII_out) -> Furnace/8(T_aII_in)
  Constant inputs/3(F_aI) -> Bus Creator7/3
  Constant inputs/2(Fw) -> Bus Creator7/2
  Bus Creator4/1 -> Multiport Switch2/2
  Bus Selector4/4 -> <Fi_aI>/1  "<Fi_aI>"
  Bus Selector4/3 -> <Fi_w>/1  "<Fi_w>"
  Bus Selector4/2 -> <Q_grate>/1  "<Q_grate>"
  Bus Selector4/1 -> <v_grate>/1  "<v_grate>"

== system Furnace/Plant2 ==
  v_grate_in : Inport
  Q_grate_in : Inport  Port=2
  Fi_w_in : Inport  Port=3
  Fi_aI_in : Inport  Port=4
  T_w_in : Inport  Port=5
  T_aI_in : Inport  Port=6
  F_aII_in : Inport  Port=7
  T_aII_in : Inport  Port=8
  Ashes : Subsystem
      mask Display: image('ash.jpg');
  "Auxiliary \"burners\"" : Subsystem
      mask Display: image('burnerim.jpg');
  Boiler : Subsystem
      mask Display: image('Boiler.jpg');
  Bus Selector : BusSelector  OutputSignals=F_w_ash
  Calorific Value : Subsystem
  Cold water from district heating : Subsystem
      mask Display: image('fromdh.jpg');
  Condenser : Subsystem
      mask Display: image('Condenser.jpg');
  Flue-gas fan : Subsystem  Commented=on
      mask Display: image('Fan.jpg');
  Flue-gas stack : Subsystem  Commented=on
      mask Display: image('Stack.jpg');
  Free board : Subsystem
      mask Display: image('fbim.jpg');
  Gas cleaning systems : Subsystem  Commented=on
      mask Display: image('Cleaning.jpg');
  Grate : Subsystem
      settings: MinAlgLoopOccurrences=on
      mask Display: image('grateim.jpg');
  Hot water to district heating : Subsystem
      mask Display: image('todh.jpg');
  Scope : Scope
  Scope1 : Scope
  Scope2 : Scope
  Turbine : Subsystem
      mask Display: image('Turbine.jpg');
  HHV_out : Outport  VectorParamsAs1DForOutWhenUnconnected=off
  F_fg_out : Outport  Port=2  VectorParamsAs1DForOutWhenUnconnected=off
  F_st_out : Outport  Port=3  VectorParamsAs1DForOutWhenUnconnected=off
  wires:
  Boiler/3(p_drum) -> Turbine/3(p_drum)
  Free board/1(T_fg_out) -> Calorific Value/1(T_fg), Scope/1, Boiler/2(T_fg), Grate/1(T_rad), "Auxiliary \"burners\""/1(In1)  "T_rad"
  Turbine/1(F_turb) -> Condenser/2(F_turb)
  Grate/1(Fi_fg_from_grate) -> Ashes/1(In1), Free board/1(Fi_in)
  Q_grate_in/1 -> Grate/4(Q_grate)
  Condenser/1(T_district) -> Hot water to district heating/1(In1)
  Cold water from district heating/1(Out1) -> Condenser/1(F_district)
  Grate/2(T_w_grate) -> Ashes/2(In2), Free board/2(T_in)
  "Auxiliary \"burners\""/1(Out1) -> Scope1/1, Grate/2(Q_burners)  "Q_burners"
  Grate/4(Q_rad_fg) -> Free board/3(Q_rad)
  Free board/2(Fi_fg_to_boiler) -> F_fg_out/1, Calorific Value/2(Fi_fg), Boiler/3(F_fg)
  Flue-gas fan/1(Out1) -> Flue-gas stack/1(T_fg)
  Boiler/4(T_fg_out) -> Gas cleaning systems/1(T_fg)
  Boiler/2(F_SH) -> Turbine/2(F_SH), F_st_out/1  "F_steam"
  Flue-gas fan/2(Out2) -> Flue-gas stack/2(Fi_fg)
  Grate/5(OutBus) -> Bus Selector/1, Ashes/3(InBus)
  Condenser/2(T_w_out) -> Boiler/1(T_fromHE)
  Gas cleaning systems/2(Fi_fg_clean) -> Flue-gas fan/2(Fi_fg)
  Boiler/1(T_SH) -> Turbine/1(T_SH)
  Free board/3(F_flyash_tot) -> Boiler/4(F_flyash)
  Grate/3(F_flyash) -> Free board/4(F_flyash_cell)
  Gas cleaning systems/1(T_fg_clean) -> Flue-gas fan/1(T_fg)
  v_grate_in/1 -> Grate/3(v_grate_in)
  Boiler/5(Fi_fg_out) -> Gas cleaning systems/2(F_fg)
  Condenser/3(F_cond) -> Boiler/5(F_ECO)
  Boiler/6(F_flyash_out) -> Gas cleaning systems/3(F_flyash)
  Cold water from district heating/2(Out2) -> Condenser/3(T_return)
  Calorific Value/1(HHV) -> HHV_out/1  "HHV"
  Fi_w_in/1 -> Grate/5(Fi_w_in)
  Fi_aI_in/1 -> Grate/6(F_aI_in)
  T_w_in/1 -> Grate/7(T_w_in)
  T_aI_in/1 -> Grate/8(T_aI_in)
  F_aII_in/1 -> Free board/5(F_aII_in)
  T_aII_in/1 -> Free board/6(T_aII_in)
  Bus Selector/1 -> Scope2/1  "<F_w_ash>"

== system Furnace/Actuator dynamics/Grate speed ==
  v_grate_reg_in : Inport
  Constant : Constant  Value=reg.const_Q_grate
  Constant1 : Constant  Value=reg.input_type_v_grate
  Constant2 : Constant  Value=reg.input_type_Q_grate
  From Workspace2 : FromWorkspace  VariableName=Q_grate
  Input  selector : MATLAB Function  TreatAsAtomicUnit=on
  Input  selector1 : MATLAB Function  TreatAsAtomicUnit=on
  Step1 : Step  Time=reg.stepTime  Before=reg.const_Q_grate  After=reg.const_Q_grate_post_step  SampleTime=0
  Step2 : Step  Time=reg.stepTime  Before=reg.const_v_grate  After=reg.const_v_grate_post_step  SampleTime=0
  To Workspace5 : ToWorkspace  VariableName=simout_v_grate  SaveFormat=Timeseries  SampleTime=-1
  const_Q_grate : Constant  Value=reg.const_Q_grate
  const_v_grate : Constant  Value=reg.const_v_grate
  v_grate : Constant  Value=k.v_grate
  v_grate_out : Outport  VectorParamsAs1DForOutWhenUnconnected=off
  Q_grate_out : Outport  Port=2  VectorParamsAs1DForOutWhenUnconnected=off
  u_v_grate : Outport  Port=3  VectorParamsAs1DForOutWhenUnconnected=off
  wires:
  v_grate/1 -> Input  selector/2(experimental)
  Input  selector/1(signal) -> To Workspace5/1, u_v_grate/1, v_grate_out/1  "v_grate"
  Constant1/1 -> Input  selector/5(input_type)
  v_grate_reg_in/1 -> Input  selector/4(controlled)
  const_v_grate/1 -> Input  selector/1(constant)  "const_v_grate"
  const_Q_grate/1 -> Input  selector1/1(constant)  "const_Q_grate"
  Constant2/1 -> Input  selector1/5(input_type)
  Input  selector1/1(signal) -> Q_grate_out/1  "Q_grate"
  From Workspace2/1 -> Input  selector1/2(experimental)
  Constant/1 -> Input  selector1/4(controlled)
  Step1/1 -> Input  selector1/3(step)  "Step"
  Step2/1 -> Input  selector/3(step)  "Step"

== system Furnace/Actuator dynamics/Secondary air ==
  F_aII_reg_in : Inport
  Constant : Constant  Value=reg.input_type_F_aII
  Constant2 : Constant  Value=reg.const_T_aII
  Constant3 : Constant  Value=reg.input_type_T_aII
  Flue gas fan : Subsystem
  From Workspace1 : FromWorkspace  VariableName=F_aII
  Input  selector : MATLAB Function  TreatAsAtomicUnit=on
  Input  selector1 : MATLAB Function  TreatAsAtomicUnit=on
  PID Controller : simulink/Continuous/PID Controller  Controller=PI  Form=Parallel  TimeDomain=Continuous-time  UseExternalTs=off  SampleTime=1  IntegratorMethod=Forward Euler  FilterMethod=Forward Euler  ControllerParametersSource=internal  P=reg.Kp_fan  I=reg.Ki_fan  D=0  UseFilter=on  N=100  TunerSelectOption=Transfer Function Based (PID Tuner App)  InitialConditionSource=internal  InitialConditionForIntegrator=reg.F_aII_fan_PID_int  InitialConditionForFilter=0  DifferentiatorICPrevScaledInput=0  ExternalReset=none  TrackingMode=off  Kt=1  LimitOutput=off  UpperSaturationLimit=inf  LowerSaturationLimit=-inf  LinearizeAsGain=on  AntiWindupMode=none  Kb=1  POutMin=[]  POutMax=[]  IOutMin=[]  IOutMax=[]  DOutMin=[]  DOutMax=[]  NOutMin=[]  NOutMax=[]  SumOutMin=[]  SumOutMax=[]  SaturationOutMin=[]  SaturationOutMax=[]  PParamMin=[]  PParamMax=[]  IParamMin=[]  IParamMax=[]  DParamMin=[]  DParamMax=[]  NParamMin=[]  NParamMax=[]  KbParamMin=[]  KbParamMax=[]  KtParamMin=[]  KtParamMax=[]  KbOutMin=[]  KbOutMax=[]  KtOutMin=[]  KtOutMax=[]  IntegratorOutMin=[]  IntegratorOutMax=[]  FilterOutMin=[]  FilterOutMax=[]  SumI1OutMin=[]  SumI1OutMax=[]  SumI2OutMin=[]  SumI2OutMax=[]  SumI3OutMin=[]  SumI3OutMax=[]  SumI4OutMin=[]  SumI4OutMax=[]  SumDOutMin=[]  SumDOutMax=[]  DifferentiatorOutMin=[]  DifferentiatorOutMax=[]  FilterDiffOutCoefMin=[]  FilterDiffOutCoefMax=[]  ReciprocalOutMin=[]  ReciprocalOutMax=[]  SumDenOutMin=[]  SumDenOutMax=[]  SumNumOutMin=[]  SumNumOutMax=[]  DivideOutMin=[]  DivideOutMax=[]  UdiffTsProdOutMin=[]  UdiffTsProdOutMax=[]  NTsProdOutMin=[]  NTsProdOutMax=[]  UintegralTsProdOutMin=[]  UintegralTsProdOutMax=[]  UngainTsProdOutMin=[]  UngainTsProdOutMax=[]  IntegratorContinuousStateAttributes=''  IntegratorStateMustResolveToSignalObject=off  IntegratorRTWStateStorageClass=Auto  FilterContinuousStateAttributes=''  FilterStateMustResolveToSignalObject=off  FilterRTWStateStorageClass=Auto  ParallelPVariant=InternalParameters  IdealPVariant=Disabled  IVariant=InternalParameters  DVariant=Disabled  IntegratorVariant=Continuous  SatVariant=Disabled  AWVariant=Passthrough  PCopyVariant=Disabled  TRVariant=Disabled  FdbkBlocksVariant=Forward  IdealPFdbkVariant=Disabled  SatFdbkVariant=Disabled  DerivativeFilterVariant=Disabled  NVariant=Disabled  NCopyVariant=Disabled_SignalSpec  FilterICVariant=Disabled  IntegratorICVariant=InternalICs  ExternalResetVariant=Disabled  TRSumVariant=Passthrough  SumFdbkVariant=Disabled  SumVariant=Sum_PI  TsampFilterVariant=InternalTs  TsampNgainVariant=Passthrough  TsampIntegralVariant=Passthrough
  Step : Step  Time=reg.stepTime  Before=reg.const_F_aII  After=reg.const_F_aII_post_step  SampleTime=0
  Step1 : Step  Time=reg.stepTime  Before=reg.const_T_aII  After=reg.const_T_aII_post_step  SampleTime=0
  Sum1 : Sum  Inputs=|+-
  T_aII : FromWorkspace  VariableName=T_aII
  To Workspace3 : ToWorkspace  VariableName=simout_F_aII  SaveFormat=Timeseries  SampleTime=-1
  const_F_aII : Constant  Value=reg.const_F_aII
  F_aII_out : Outport  VectorParamsAs1DForOutWhenUnconnected=off
  T_aII_out : Outport  Port=2  VectorParamsAs1DForOutWhenUnconnected=off
  u_F_aII : Outport  Port=3  VectorParamsAs1DForOutWhenUnconnected=off
  tag scope: F_aII=global, T_aII=global
  wires:
  Constant2/1 -> Input  selector1/1(constant)
  T_aII/1 -> Input  selector1/2(experimental)
  From Workspace1/1 -> Input  selector/2(experimental)
  const_F_aII/1 -> Input  selector/1(constant)  "const_F_aII"
  Constant/1 -> Input  selector/5(input_type)
  Constant3/1 -> Input  selector1/5(input_type)
  Input  selector1/1(signal) -> T_aII_out/1, [T_aII]
  Sum1/1 -> PID Controller/1
  PID Controller/1 -> Flue gas fan/1(PID signal)
  Input  selector/1(signal) -> To Workspace3/1, u_F_aII/1, Sum1/1  "F_aII"
  Flue gas fan/1(Volume flow) -> [F_aII], F_aII_out/1, Sum1/2
  Step/1 -> Input  selector/3(step)  "Step"
  F_aII_reg_in/1 -> Input  selector/4(controlled)
  Step1/1 -> Input  selector1/3(step)  "Step"
